simulink model "Teste"  (R2020b)
settings: Solver=VariableStepAuto  StartTime=0.0  StopTime=10.0  RelTol=1e-3
undefined symbols (not defined in the file or in its folder): des, SELECT, T
libraries: simulink x8
(part 2 of 3)

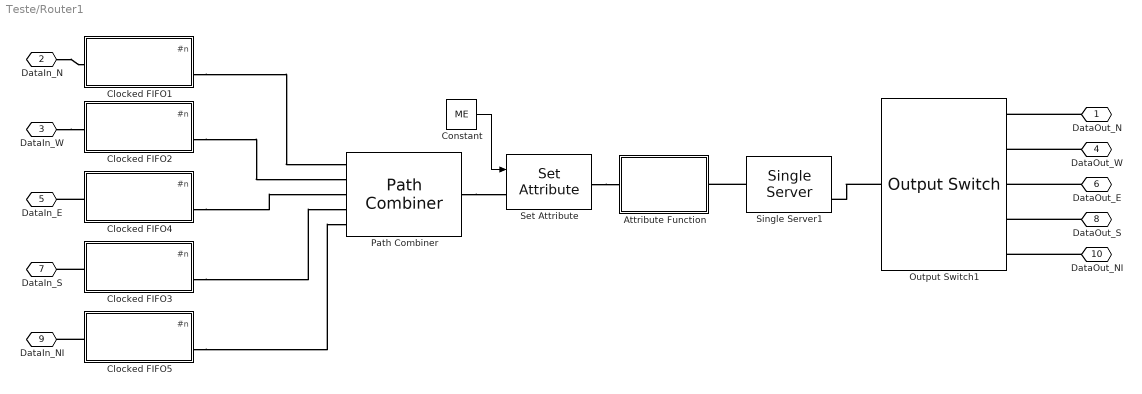
== system Teste/Router1 ==
  Attribute Function : Subsystem  LoadFcn=des.afb.attributefunction_support(gcb,'LoadFcn');  StartFcn=des.afb.attributefunction_support(gcb,'StartFcn');  mask(Attribute Function){OutputNamePrefix=out_}
      mask prompts: OutputNamePrefix "Prefix name"
      settings: CopyFcn=des.afb.attributefunction_support(gcb,'CopyFcn');  OpenFcn=des.afb.attributefunction_support(gcb,'OpenFcn');  ErrorFcn=des.afb.error_redirect
      mask Help: slhelp(gcbh)
      mask Display: image(des_iconLoad('attribFunction.jpg'),'center');
  Clocked FIFO1 : Subsystem  mask{E=1/F, S=S, F=C}
      mask prompts: E "Clock Period (s)"; S "Standard Deviation"; F "FIFO capacity"
  Clocked FIFO2 : Subsystem  mask{E=1, S=.1, F=8}
      mask prompts: E "Clock Period (s)"; S "Standard Deviation"; F "FIFO capacity"
  Clocked FIFO3 : Subsystem  mask{E=1, S=.1, F=8}
      mask prompts: E "Clock Period (s)"; S "Standard Deviation"; F "FIFO capacity"
  Clocked FIFO4 : Subsystem  mask{E=1, S=.1, F=8}
      mask prompts: E "Clock Period (s)"; S "Standard Deviation"; F "FIFO capacity"
  Clocked FIFO5 : Subsystem  mask{E=1, S=.1, F=8}
      mask prompts: E "Clock Period (s)"; S "Standard Deviation"; F "FIFO capacity"
  Constant : Constant  Value=ME
  Output Switch1 : OutputSwitch  NumberOutputPorts=5  SwitchingCriterion=From attribute  AttributeName=RT  InitialConditionsOpt=on  InitialConditions=5
  Path Combiner : PathCombiner  NumberInputPorts=5  InputPortPrecedence=Equiprobable  InitialSeed=2
  Set Attribute : SetAttribute  AttributeName=ME  AttributeFrom=Signal port  EvaluatedAttributeValue={ []}
  Single Server1 : SingleServer  ServiceTime=D  StatNumberDeparted=on
  DataOut_N : PMIOPort  Side=Left
  DataIn_N : PMIOPort  Port=2  Side=Right
  DataIn_W : PMIOPort  Port=3  Side=Left
  DataOut_W : PMIOPort  Port=4  Side=Right
  DataIn_E : PMIOPort  Port=5  Side=Left
  DataOut_E : PMIOPort  Port=6  Side=Right
  DataIn_S : PMIOPort  Port=7  Side=Left
  DataOut_S : PMIOPort  Port=8  Side=Right
  DataIn_NI : PMIOPort  Port=9  Side=Left
  DataOut_NI : PMIOPort  Port=10  Side=Right
  wires:
  Constant/1 -> Set Attribute/1
  connections:
  DataOut_NI/RConn1 -- Output Switch1/RConn5
  DataOut_S/RConn1 -- Output Switch1/RConn4
  DataOut_E/RConn1 -- Output Switch1/RConn3
  DataOut_W/RConn1 -- Output Switch1/RConn2
  DataOut_N/RConn1 -- Output Switch1/RConn1
  Clocked FIFO5/RConn1 -- Path Combiner/LConn5
  Clocked FIFO3/RConn1 -- Path Combiner/LConn4
  Clocked FIFO4/RConn1 -- Path Combiner/LConn3
  Clocked FIFO2/RConn1 -- Path Combiner/LConn2
  Clocked FIFO1/RConn1 -- Path Combiner/LConn1
  Path Combiner/RConn1 -- Set Attribute/LConn1
  Single Server1/LConn1 -- Attribute Function/RConn1
  Output Switch1/LConn1 -- Single Server1/RConn1
  Set Attribute/RConn1 -- Attribute Function/LConn1
  Clocked FIFO5/LConn1 -- DataIn_NI/RConn1
  DataIn_N/RConn1 -- Clocked FIFO1/LConn1
  Clocked FIFO3/LConn1 -- DataIn_S/RConn1
  Clocked FIFO4/LConn1 -- DataIn_E/RConn1
  DataIn_W/RConn1 -- Clocked FIFO2/LConn1

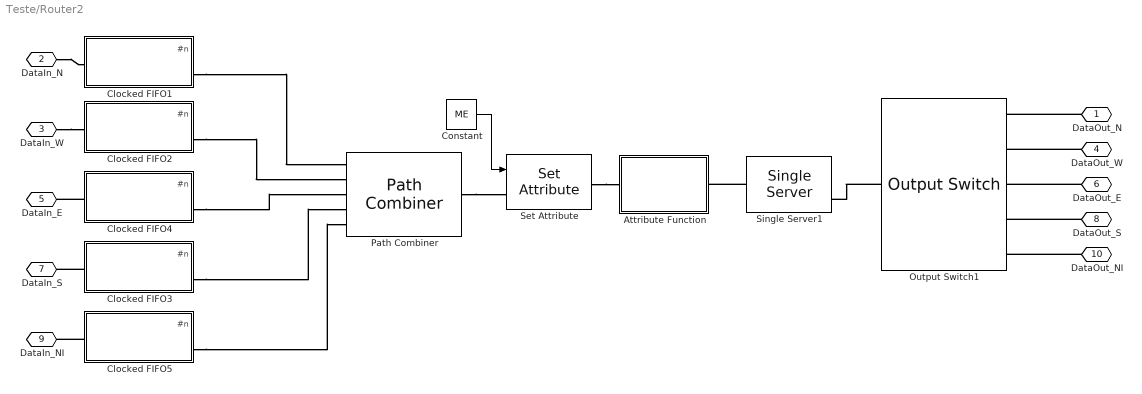
== system Teste/Router2 ==
  Attribute Function : Subsystem  LoadFcn=des.afb.attributefunction_support(gcb,'LoadFcn');  StartFcn=des.afb.attributefunction_support(gcb,'StartFcn');  mask(Attribute Function){OutputNamePrefix=out_}
      mask prompts: OutputNamePrefix "Prefix name"
      settings: CopyFcn=des.afb.attributefunction_support(gcb,'CopyFcn');  OpenFcn=des.afb.attributefunction_support(gcb,'OpenFcn');  ErrorFcn=des.afb.error_redirect
      mask Help: slhelp(gcbh)
      mask Display: image(des_iconLoad('attribFunction.jpg'),'center');
  Clocked FIFO1 : Subsystem  mask{E=1/F, S=S, F=C}
      mask prompts: E "Clock Period (s)"; S "Standard Deviation"; F "FIFO capacity"
  Clocked FIFO2 : Subsystem  mask{E=1, S=.1, F=8}
      mask prompts: E "Clock Period (s)"; S "Standard Deviation"; F "FIFO capacity"
  Clocked FIFO3 : Subsystem  mask{E=1, S=.1, F=8}
      mask prompts: E "Clock Period (s)"; S "Standard Deviation"; F "FIFO capacity"
  Clocked FIFO4 : Subsystem  mask{E=1, S=.1, F=8}
      mask prompts: E "Clock Period (s)"; S "Standard Deviation"; F "FIFO capacity"
  Clocked FIFO5 : Subsystem  mask{E=1, S=.1, F=8}
      mask prompts: E "Clock Period (s)"; S "Standard Deviation"; F "FIFO capacity"
  Constant : Constant  Value=ME
  Output Switch1 : OutputSwitch  NumberOutputPorts=5  SwitchingCriterion=From attribute  AttributeName=RT  InitialConditionsOpt=on  InitialConditions=5
  Path Combiner : PathCombiner  NumberInputPorts=5  InputPortPrecedence=Equiprobable  InitialSeed=2
  Set Attribute : SetAttribute  AttributeName=ME  AttributeFrom=Signal port  EvaluatedAttributeValue={ []}
  Single Server1 : SingleServer  ServiceTime=D  StatNumberDeparted=on
  DataOut_N : PMIOPort  Side=Left
  DataIn_N : PMIOPort  Port=2  Side=Right
  DataIn_W : PMIOPort  Port=3  Side=Left
  DataOut_W : PMIOPort  Port=4  Side=Right
  DataIn_E : PMIOPort  Port=5  Side=Left
  DataOut_E : PMIOPort  Port=6  Side=Right
  DataIn_S : PMIOPort  Port=7  Side=Left
  DataOut_S : PMIOPort  Port=8  Side=Right
  DataIn_NI : PMIOPort  Port=9  Side=Left
  DataOut_NI : PMIOPort  Port=10  Side=Right
  wires:
  Constant/1 -> Set Attribute/1
  connections:
  DataOut_NI/RConn1 -- Output Switch1/RConn5
  DataOut_S/RConn1 -- Output Switch1/RConn4
  DataOut_E/RConn1 -- Output Switch1/RConn3
  DataOut_W/RConn1 -- Output Switch1/RConn2
  DataOut_N/RConn1 -- Output Switch1/RConn1
  Clocked FIFO5/RConn1 -- Path Combiner/LConn5
  Clocked FIFO3/RConn1 -- Path Combiner/LConn4
  Clocked FIFO4/RConn1 -- Path Combiner/LConn3
  Clocked FIFO2/RConn1 -- Path Combiner/LConn2
  Clocked FIFO1/RConn1 -- Path Combiner/LConn1
  Path Combiner/RConn1 -- Set Attribute/LConn1
  Single Server1/LConn1 -- Attribute Function/RConn1
  Output Switch1/LConn1 -- Single Server1/RConn1
  Set Attribute/RConn1 -- Attribute Function/LConn1
  Clocked FIFO5/LConn1 -- DataIn_NI/RConn1
  DataIn_N/RConn1 -- Clocked FIFO1/LConn1
  Clocked FIFO3/LConn1 -- DataIn_S/RConn1
  Clocked FIFO4/LConn1 -- DataIn_E/RConn1
  DataIn_W/RConn1 -- Clocked FIFO2/LConn1

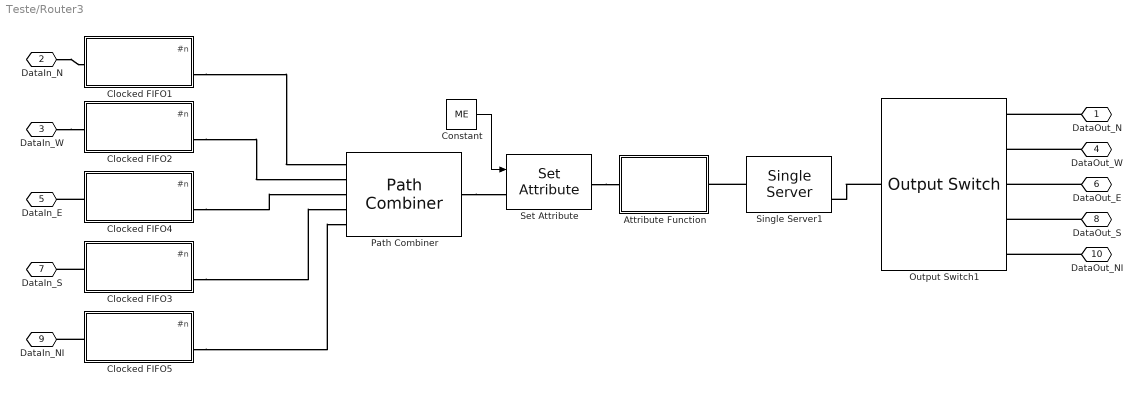
== system Teste/Router3 ==
  Attribute Function : Subsystem  LoadFcn=des.afb.attributefunction_support(gcb,'LoadFcn');  StartFcn=des.afb.attributefunction_support(gcb,'StartFcn');  mask(Attribute Function){OutputNamePrefix=out_}
      mask prompts: OutputNamePrefix "Prefix name"
      settings: CopyFcn=des.afb.attributefunction_support(gcb,'CopyFcn');  OpenFcn=des.afb.attributefunction_support(gcb,'OpenFcn');  ErrorFcn=des.afb.error_redirect
      mask Help: slhelp(gcbh)
      mask Display: image(des_iconLoad('attribFunction.jpg'),'center');
  Clocked FIFO1 : Subsystem  mask{E=1/F, S=S, F=C}
      mask prompts: E "Clock Period (s)"; S "Standard Deviation"; F "FIFO capacity"
  Clocked FIFO2 : Subsystem  mask{E=1, S=.1, F=8}
      mask prompts: E "Clock Period (s)"; S "Standard Deviation"; F "FIFO capacity"
  Clocked FIFO3 : Subsystem  mask{E=1, S=.1, F=8}
      mask prompts: E "Clock Period (s)"; S "Standard Deviation"; F "FIFO capacity"
  Clocked FIFO4 : Subsystem  mask{E=1, S=.1, F=8}
      mask prompts: E "Clock Period (s)"; S "Standard Deviation"; F "FIFO capacity"
  Clocked FIFO5 : Subsystem  mask{E=1, S=.1, F=8}
      mask prompts: E "Clock Period (s)"; S "Standard Deviation"; F "FIFO capacity"
  Constant : Constant  Value=ME
  Output Switch1 : OutputSwitch  NumberOutputPorts=5  SwitchingCriterion=From attribute  AttributeName=RT  InitialConditionsOpt=on  InitialConditions=5
  Path Combiner : PathCombiner  NumberInputPorts=5  InputPortPrecedence=Equiprobable  InitialSeed=2
  Set Attribute : SetAttribute  AttributeName=ME  AttributeFrom=Signal port  EvaluatedAttributeValue={ []}
  Single Server1 : SingleServer  ServiceTime=D  StatNumberDeparted=on
  DataOut_N : PMIOPort  Side=Left
  DataIn_N : PMIOPort  Port=2  Side=Right
  DataIn_W : PMIOPort  Port=3  Side=Left
  DataOut_W : PMIOPort  Port=4  Side=Right
  DataIn_E : PMIOPort  Port=5  Side=Left
  DataOut_E : PMIOPort  Port=6  Side=Right
  DataIn_S : PMIOPort  Port=7  Side=Left
  DataOut_S : PMIOPort  Port=8  Side=Right
  DataIn_NI : PMIOPort  Port=9  Side=Left
  DataOut_NI : PMIOPort  Port=10  Side=Right
  wires:
  Constant/1 -> Set Attribute/1
  connections:
  DataOut_NI/RConn1 -- Output Switch1/RConn5
  DataOut_S/RConn1 -- Output Switch1/RConn4
  DataOut_E/RConn1 -- Output Switch1/RConn3
  DataOut_W/RConn1 -- Output Switch1/RConn2
  DataOut_N/RConn1 -- Output Switch1/RConn1
  Clocked FIFO5/RConn1 -- Path Combiner/LConn5
  Clocked FIFO3/RConn1 -- Path Combiner/LConn4
  Clocked FIFO4/RConn1 -- Path Combiner/LConn3
  Clocked FIFO2/RConn1 -- Path Combiner/LConn2
  Clocked FIFO1/RConn1 -- Path Combiner/LConn1
  Path Combiner/RConn1 -- Set Attribute/LConn1
  Single Server1/LConn1 -- Attribute Function/RConn1
  Output Switch1/LConn1 -- Single Server1/RConn1
  Set Attribute/RConn1 -- Attribute Function/LConn1
  Clocked FIFO5/LConn1 -- DataIn_NI/RConn1
  DataIn_N/RConn1 -- Clocked FIFO1/LConn1
  Clocked FIFO3/LConn1 -- DataIn_S/RConn1
  Clocked FIFO4/LConn1 -- DataIn_E/RConn1
  DataIn_W/RConn1 -- Clocked FIFO2/LConn1

== system Teste/Router4 ==
  Attribute Function : Subsystem  LoadFcn=des.afb.attributefunction_support(gcb,'LoadFcn');  StartFcn=des.afb.attributefunction_support(gcb,'StartFcn');  mask(Attribute Function){OutputNamePrefix=out_}
      mask prompts: OutputNamePrefix "Prefix name"
      settings: CopyFcn=des.afb.attributefunction_support(gcb,'CopyFcn');  OpenFcn=des.afb.attributefunction_support(gcb,'OpenFcn');  ErrorFcn=des.afb.error_redirect
      mask Help: slhelp(gcbh)
      mask Display: image(des_iconLoad('attribFunction.jpg'),'center');
  Clocked FIFO1 : Subsystem  mask{E=1/F, S=S, F=C}
      mask prompts: E "Clock Period (s)"; S "Standard Deviation"; F "FIFO capacity"
  Clocked FIFO2 : Subsystem  mask{E=1, S=.1, F=8}
      mask prompts: E "Clock Period (s)"; S "Standard Deviation"; F "FIFO capacity"
  Clocked FIFO3 : Subsystem  mask{E=1, S=.1, F=8}
      mask prompts: E "Clock Period (s)"; S "Standard Deviation"; F "FIFO capacity"
  Clocked FIFO4 : Subsystem  mask{E=1, S=.1, F=8}
      mask prompts: E "Clock Period (s)"; S "Standard Deviation"; F "FIFO capacity"
  Clocked FIFO5 : Subsystem  mask{E=1, S=.1, F=8}
      mask prompts: E "Clock Period (s)"; S "Standard Deviation"; F "FIFO capacity"
  Constant : Constant  Value=ME
  Output Switch1 : OutputSwitch  NumberOutputPorts=5  SwitchingCriterion=From attribute  AttributeName=RT  InitialConditionsOpt=on  InitialConditions=5
  Path Combiner : PathCombiner  NumberInputPorts=5  InputPortPrecedence=Equiprobable  InitialSeed=2
  Set Attribute : SetAttribute  AttributeName=ME  AttributeFrom=Signal port  EvaluatedAttributeValue={ []}
  Single Server1 : SingleServer  ServiceTime=D  StatNumberDeparted=on
  DataOut_N : PMIOPort  Side=Left
  DataIn_N : PMIOPort  Port=2  Side=Right
  DataIn_W : PMIOPort  Port=3  Side=Left
  DataOut_W : PMIOPort  Port=4  Side=Right
  DataIn_E : PMIOPort  Port=5  Side=Left
  DataOut_E : PMIOPort  Port=6  Side=Right
  DataIn_S : PMIOPort  Port=7  Side=Left
  DataOut_S : PMIOPort  Port=8  Side=Right
  DataIn_NI : PMIOPort  Port=9  Side=Left
  DataOut_NI : PMIOPort  Port=10  Side=Right
  wires:
  Constant/1 -> Set Attribute/1
  connections:
  DataOut_NI/RConn1 -- Output Switch1/RConn5
  DataOut_S/RConn1 -- Output Switch1/RConn4
  DataOut_E/RConn1 -- Output Switch1/RConn3
  DataOut_W/RConn1 -- Output Switch1/RConn2
  DataOut_N/RConn1 -- Output Switch1/RConn1
  Clocked FIFO5/RConn1 -- Path Combiner/LConn5
  Clocked FIFO3/RConn1 -- Path Combiner/LConn4
  Clocked FIFO4/RConn1 -- Path Combiner/LConn3
  Clocked FIFO2/RConn1 -- Path Combiner/LConn2
  Clocked FIFO1/RConn1 -- Path Combiner/LConn1
  Path Combiner/RConn1 -- Set Attribute/LConn1
  Single Server1/LConn1 -- Attribute Function/RConn1
  Output Switch1/LConn1 -- Single Server1/RConn1
  Set Attribute/RConn1 -- Attribute Function/LConn1
  Clocked FIFO5/LConn1 -- DataIn_NI/RConn1
  DataIn_N/RConn1 -- Clocked FIFO1/LConn1
  Clocked FIFO3/LConn1 -- DataIn_S/RConn1
  Clocked FIFO4/LConn1 -- DataIn_E/RConn1
  DataIn_W/RConn1 -- Clocked FIFO2/LConn1

== system Teste/Router5 ==
  Attribute Function : Subsystem  LoadFcn=des.afb.attributefunction_support(gcb,'LoadFcn');  StartFcn=des.afb.attributefunction_support(gcb,'StartFcn');  mask(Attribute Function){OutputNamePrefix=out_}
      mask prompts: OutputNamePrefix "Prefix name"
      settings: CopyFcn=des.afb.attributefunction_support(gcb,'CopyFcn');  OpenFcn=des.afb.attributefunction_support(gcb,'OpenFcn');  ErrorFcn=des.afb.error_redirect
      mask Help: slhelp(gcbh)
      mask Display: image(des_iconLoad('attribFunction.jpg'),'center');
  Clocked FIFO1 : Subsystem  mask{E=1/F, S=S, F=C}
      mask prompts: E "Clock Period (s)"; S "Standard Deviation"; F "FIFO capacity"
  Clocked FIFO2 : Subsystem  mask{E=1, S=.1, F=8}
      mask prompts: E "Clock Period (s)"; S "Standard Deviation"; F "FIFO capacity"
  Clocked FIFO3 : Subsystem  mask{E=1, S=.1, F=8}
      mask prompts: E "Clock Period (s)"; S "Standard Deviation"; F "FIFO capacity"
  Clocked FIFO4 : Subsystem  mask{E=1, S=.1, F=8}
      mask prompts: E "Clock Period (s)"; S "Standard Deviation"; F "FIFO capacity"
  Clocked FIFO5 : Subsystem  mask{E=1, S=.1, F=8}
      mask prompts: E "Clock Period (s)"; S "Standard Deviation"; F "FIFO capacity"
  Constant : Constant  Value=ME
  Output Switch1 : OutputSwitch  NumberOutputPorts=5  SwitchingCriterion=From attribute  AttributeName=RT  InitialConditionsOpt=on  InitialConditions=5
  Path Combiner : PathCombiner  NumberInputPorts=5  InputPortPrecedence=Equiprobable  InitialSeed=2
  Set Attribute : SetAttribute  AttributeName=ME  AttributeFrom=Signal port  EvaluatedAttributeValue={ []}
  Single Server1 : SingleServer  ServiceTime=D  StatNumberDeparted=on
  DataOut_N : PMIOPort  Side=Left
  DataIn_N : PMIOPort  Port=2  Side=Right
  DataIn_W : PMIOPort  Port=3  Side=Left
  DataOut_W : PMIOPort  Port=4  Side=Right
  DataIn_E : PMIOPort  Port=5  Side=Left
  DataOut_E : PMIOPort  Port=6  Side=Right
  DataIn_S : PMIOPort  Port=7  Side=Left
  DataOut_S : PMIOPort  Port=8  Side=Right
  DataIn_NI : PMIOPort  Port=9  Side=Left
  DataOut_NI : PMIOPort  Port=10  Side=Right
  wires:
  Constant/1 -> Set Attribute/1
  connections:
  DataOut_NI/RConn1 -- Output Switch1/RConn5
  DataOut_S/RConn1 -- Output Switch1/RConn4
  DataOut_E/RConn1 -- Output Switch1/RConn3
  DataOut_W/RConn1 -- Output Switch1/RConn2
  DataOut_N/RConn1 -- Output Switch1/RConn1
  Clocked FIFO5/RConn1 -- Path Combiner/LConn5
  Clocked FIFO3/RConn1 -- Path Combiner/LConn4
  Clocked FIFO4/RConn1 -- Path Combiner/LConn3
  Clocked FIFO2/RConn1 -- Path Combiner/LConn2
  Clocked FIFO1/RConn1 -- Path Combiner/LConn1
  Path Combiner/RConn1 -- Set Attribute/LConn1
  Single Server1/LConn1 -- Attribute Function/RConn1
  Output Switch1/LConn1 -- Single Server1/RConn1
  Set Attribute/RConn1 -- Attribute Function/LConn1
  Clocked FIFO5/LConn1 -- DataIn_NI/RConn1
  DataIn_N/RConn1 -- Clocked FIFO1/LConn1
  Clocked FIFO3/LConn1 -- DataIn_S/RConn1
  Clocked FIFO4/LConn1 -- DataIn_E/RConn1
  DataIn_W/RConn1 -- Clocked FIFO2/LConn1

== system Teste/Router6 ==
  Attribute Function : Subsystem  LoadFcn=des.afb.attributefunction_support(gcb,'LoadFcn');  StartFcn=des.afb.attributefunction_support(gcb,'StartFcn');  mask(Attribute Function){OutputNamePrefix=out_}
      mask prompts: OutputNamePrefix "Prefix name"
      settings: CopyFcn=des.afb.attributefunction_support(gcb,'CopyFcn');  OpenFcn=des.afb.attributefunction_support(gcb,'OpenFcn');  ErrorFcn=des.afb.error_redirect
      mask Help: slhelp(gcbh)
      mask Display: image(des_iconLoad('attribFunction.jpg'),'center');
  Clocked FIFO1 : Subsystem  mask{E=1/F, S=S, F=C}
      mask prompts: E "Clock Period (s)"; S "Standard Deviation"; F "FIFO capacity"
  Clocked FIFO2 : Subsystem  mask{E=1, S=.1, F=8}
      mask prompts: E "Clock Period (s)"; S "Standard Deviation"; F "FIFO capacity"
  Clocked FIFO3 : Subsystem  mask{E=1, S=.1, F=8}
      mask prompts: E "Clock Period (s)"; S "Standard Deviation"; F "FIFO capacity"
  Clocked FIFO4 : Subsystem  mask{E=1, S=.1, F=8}
      mask prompts: E "Clock Period (s)"; S "Standard Deviation"; F "FIFO capacity"
  Clocked FIFO5 : Subsystem  mask{E=1, S=.1, F=8}
      mask prompts: E "Clock Period (s)"; S "Standard Deviation"; F "FIFO capacity"
  Constant : Constant  Value=ME
  Output Switch1 : OutputSwitch  NumberOutputPorts=5  SwitchingCriterion=From attribute  AttributeName=RT  InitialConditionsOpt=on  InitialConditions=5
  Path Combiner : PathCombiner  NumberInputPorts=5  InputPortPrecedence=Equiprobable  InitialSeed=2
  Set Attribute : SetAttribute  AttributeName=ME  AttributeFrom=Signal port  EvaluatedAttributeValue={ []}
  Single Server1 : SingleServer  ServiceTime=D  StatNumberDeparted=on
  DataOut_N : PMIOPort  Side=Left
  DataIn_N : PMIOPort  Port=2  Side=Right
  DataIn_W : PMIOPort  Port=3  Side=Left
  DataOut_W : PMIOPort  Port=4  Side=Right
  DataIn_E : PMIOPort  Port=5  Side=Left
  DataOut_E : PMIOPort  Port=6  Side=Right
  DataIn_S : PMIOPort  Port=7  Side=Left
  DataOut_S : PMIOPort  Port=8  Side=Right
  DataIn_NI : PMIOPort  Port=9  Side=Left
  DataOut_NI : PMIOPort  Port=10  Side=Right
  wires:
  Constant/1 -> Set Attribute/1
  connections:
  DataOut_NI/RConn1 -- Output Switch1/RConn5
  DataOut_S/RConn1 -- Output Switch1/RConn4
  DataOut_E/RConn1 -- Output Switch1/RConn3
  DataOut_W/RConn1 -- Output Switch1/RConn2
  DataOut_N/RConn1 -- Output Switch1/RConn1
  Clocked FIFO5/RConn1 -- Path Combiner/LConn5
  Clocked FIFO3/RConn1 -- Path Combiner/LConn4
  Clocked FIFO4/RConn1 -- Path Combiner/LConn3
  Clocked FIFO2/RConn1 -- Path Combiner/LConn2
  Clocked FIFO1/RConn1 -- Path Combiner/LConn1
  Path Combiner/RConn1 -- Set Attribute/LConn1
  Single Server1/LConn1 -- Attribute Function/RConn1
  Output Switch1/LConn1 -- Single Server1/RConn1
  Set Attribute/RConn1 -- Attribute Function/LConn1
  Clocked FIFO5/LConn1 -- DataIn_NI/RConn1
  DataIn_N/RConn1 -- Clocked FIFO1/LConn1
  Clocked FIFO3/LConn1 -- DataIn_S/RConn1
  Clocked FIFO4/LConn1 -- DataIn_E/RConn1
  DataIn_W/RConn1 -- Clocked FIFO2/LConn1

== system Teste/Router7 ==
  Attribute Function : Subsystem  LoadFcn=des.afb.attributefunction_support(gcb,'LoadFcn');  StartFcn=des.afb.attributefunction_support(gcb,'StartFcn');  mask(Attribute Function){OutputNamePrefix=out_}
      mask prompts: OutputNamePrefix "Prefix name"
      settings: CopyFcn=des.afb.attributefunction_support(gcb,'CopyFcn');  OpenFcn=des.afb.attributefunction_support(gcb,'OpenFcn');  ErrorFcn=des.afb.error_redirect
      mask Help: slhelp(gcbh)
      mask Display: image(des_iconLoad('attribFunction.jpg'),'center');
  Clocked FIFO1 : Subsystem  mask{E=1/F, S=S, F=C}
      mask prompts: E "Clock Period (s)"; S "Standard Deviation"; F "FIFO capacity"
  Clocked FIFO2 : Subsystem  mask{E=1, S=.1, F=8}
      mask prompts: E "Clock Period (s)"; S "Standard Deviation"; F "FIFO capacity"
  Clocked FIFO3 : Subsystem  mask{E=1, S=.1, F=8}
      mask prompts: E "Clock Period (s)"; S "Standard Deviation"; F "FIFO capacity"
  Clocked FIFO4 : Subsystem  mask{E=1, S=.1, F=8}
      mask prompts: E "Clock Period (s)"; S "Standard Deviation"; F "FIFO capacity"
  Clocked FIFO5 : Subsystem  mask{E=1, S=.1, F=8}
      mask prompts: E "Clock Period (s)"; S "Standard Deviation"; F "FIFO capacity"
  Constant : Constant  Value=ME
  Output Switch1 : OutputSwitch  NumberOutputPorts=5  SwitchingCriterion=From attribute  AttributeName=RT  InitialConditionsOpt=on  InitialConditions=5
  Path Combiner : PathCombiner  NumberInputPorts=5  InputPortPrecedence=Equiprobable  InitialSeed=2
  Set Attribute : SetAttribute  AttributeName=ME  AttributeFrom=Signal port  EvaluatedAttributeValue={ []}
  Single Server1 : SingleServer  ServiceTime=D  StatNumberDeparted=on
  DataOut_N : PMIOPort  Side=Left
  DataIn_N : PMIOPort  Port=2  Side=Right
  DataIn_W : PMIOPort  Port=3  Side=Left
  DataOut_W : PMIOPort  Port=4  Side=Right
  DataIn_E : PMIOPort  Port=5  Side=Left
  DataOut_E : PMIOPort  Port=6  Side=Right
  DataIn_S : PMIOPort  Port=7  Side=Left
  DataOut_S : PMIOPort  Port=8  Side=Right
  DataIn_NI : PMIOPort  Port=9  Side=Left
  DataOut_NI : PMIOPort  Port=10  Side=Right
  wires:
  Constant/1 -> Set Attribute/1
  connections:
  DataOut_NI/RConn1 -- Output Switch1/RConn5
  DataOut_S/RConn1 -- Output Switch1/RConn4
  DataOut_E/RConn1 -- Output Switch1/RConn3
  DataOut_W/RConn1 -- Output Switch1/RConn2
  DataOut_N/RConn1 -- Output Switch1/RConn1
  Clocked FIFO5/RConn1 -- Path Combiner/LConn5
  Clocked FIFO3/RConn1 -- Path Combiner/LConn4
  Clocked FIFO4/RConn1 -- Path Combiner/LConn3
  Clocked FIFO2/RConn1 -- Path Combiner/LConn2
  Clocked FIFO1/RConn1 -- Path Combiner/LConn1
  Path Combiner/RConn1 -- Set Attribute/LConn1
  Single Server1/LConn1 -- Attribute Function/RConn1
  Output Switch1/LConn1 -- Single Server1/RConn1
  Set Attribute/RConn1 -- Attribute Function/LConn1
  Clocked FIFO5/LConn1 -- DataIn_NI/RConn1
  DataIn_N/RConn1 -- Clocked FIFO1/LConn1
  Clocked FIFO3/LConn1 -- DataIn_S/RConn1
  Clocked FIFO4/LConn1 -- DataIn_E/RConn1
  DataIn_W/RConn1 -- Clocked FIFO2/LConn1

== system Teste/Router8 ==
  Attribute Function : Subsystem  LoadFcn=des.afb.attributefunction_support(gcb,'LoadFcn');  StartFcn=des.afb.attributefunction_support(gcb,'StartFcn');  mask(Attribute Function){OutputNamePrefix=out_}
      mask prompts: OutputNamePrefix "Prefix name"
      settings: CopyFcn=des.afb.attributefunction_support(gcb,'CopyFcn');  OpenFcn=des.afb.attributefunction_support(gcb,'OpenFcn');  ErrorFcn=des.afb.error_redirect
      mask Help: slhelp(gcbh)
      mask Display: image(des_iconLoad('attribFunction.jpg'),'center');
  Clocked FIFO1 : Subsystem  mask{E=1/F, S=S, F=C}
      mask prompts: E "Clock Period (s)"; S "Standard Deviation"; F "FIFO capacity"
  Clocked FIFO2 : Subsystem  mask{E=1, S=.1, F=8}
      mask prompts: E "Clock Period (s)"; S "Standard Deviation"; F "FIFO capacity"
  Clocked FIFO3 : Subsystem  mask{E=1, S=.1, F=8}
      mask prompts: E "Clock Period (s)"; S "Standard Deviation"; F "FIFO capacity"
  Clocked FIFO4 : Subsystem  mask{E=1, S=.1, F=8}
      mask prompts: E "Clock Period (s)"; S "Standard Deviation"; F "FIFO capacity"
  Clocked FIFO5 : Subsystem  mask{E=1, S=.1, F=8}
      mask prompts: E "Clock Period (s)"; S "Standard Deviation"; F "FIFO capacity"
  Constant : Constant  Value=ME
  Output Switch1 : OutputSwitch  NumberOutputPorts=5  SwitchingCriterion=From attribute  AttributeName=RT  InitialConditionsOpt=on  InitialConditions=5
  Path Combiner : PathCombiner  NumberInputPorts=5  InputPortPrecedence=Equiprobable  InitialSeed=2
  Set Attribute : SetAttribute  AttributeName=ME  AttributeFrom=Signal port  EvaluatedAttributeValue={ []}
  Single Server1 : SingleServer  ServiceTime=D  StatNumberDeparted=on
  DataOut_N : PMIOPort  Side=Left
  DataIn_N : PMIOPort  Port=2  Side=Right
  DataIn_W : PMIOPort  Port=3  Side=Left
  DataOut_W : PMIOPort  Port=4  Side=Right
  DataIn_E : PMIOPort  Port=5  Side=Left
  DataOut_E : PMIOPort  Port=6  Side=Right
  DataIn_S : PMIOPort  Port=7  Side=Left
  DataOut_S : PMIOPort  Port=8  Side=Right
  DataIn_NI : PMIOPort  Port=9  Side=Left
  DataOut_NI : PMIOPort  Port=10  Side=Right
  wires:
  Constant/1 -> Set Attribute/1
  connections:
  DataOut_NI/RConn1 -- Output Switch1/RConn5
  DataOut_S/RConn1 -- Output Switch1/RConn4
  DataOut_E/RConn1 -- Output Switch1/RConn3
  DataOut_W/RConn1 -- Output Switch1/RConn2
  DataOut_N/RConn1 -- Output Switch1/RConn1
  Clocked FIFO5/RConn1 -- Path Combiner/LConn5
  Clocked FIFO3/RConn1 -- Path Combiner/LConn4
  Clocked FIFO4/RConn1 -- Path Combiner/LConn3
  Clocked FIFO2/RConn1 -- Path Combiner/LConn2
  Clocked FIFO1/RConn1 -- Path Combiner/LConn1
  Path Combiner/RConn1 -- Set Attribute/LConn1
  Single Server1/LConn1 -- Attribute Function/RConn1
  Output Switch1/LConn1 -- Single Server1/RConn1
  Set Attribute/RConn1 -- Attribute Function/LConn1
  Clocked FIFO5/LConn1 -- DataIn_NI/RConn1
  DataIn_N/RConn1 -- Clocked FIFO1/LConn1
  Clocked FIFO3/LConn1 -- DataIn_S/RConn1
  Clocked FIFO4/LConn1 -- DataIn_E/RConn1
  DataIn_W/RConn1 -- Clocked FIFO2/LConn1

== system Teste/PE1/Create Generator Selection Variable ==
  function : TriggerPort  TriggerType=function-call  VariantControl=(inherit)
  Repeating Sequence Stair : simulink/Sources/Repeating Sequence Stair  OutValues=[0 1].'  tsamp=-1  OutMin=[]  OutMax=[]  OutDataTypeStr=float('double')  OutputDataTypeScalingMode=Specify via dialog  OutDataType=float('double')  ConRadixGroup=Best Precision: Vector-wise  OutScaling=2^-12
  Out1 : Outport
  wires:
  Repeating Sequence Stair/1 -> Out1/1

== system Teste/PE2/Create Generator Selection Variable ==
  function : TriggerPort  TriggerType=function-call  VariantControl=(inherit)
  Repeating Sequence Stair : simulink/Sources/Repeating Sequence Stair  OutValues=[0 1].'  tsamp=-1  OutMin=[]  OutMax=[]  OutDataTypeStr=float('double')  OutputDataTypeScalingMode=Specify via dialog  OutDataType=float('double')  ConRadixGroup=Best Precision: Vector-wise  OutScaling=2^-12
  Out1 : Outport
  wires:
  Repeating Sequence Stair/1 -> Out1/1

== system Teste/PE3/Create Generator Selection Variable ==
  function : TriggerPort  TriggerType=function-call  VariantControl=(inherit)
  Repeating Sequence Stair : simulink/Sources/Repeating Sequence Stair  OutValues=[0 1].'  tsamp=-1  OutMin=[]  OutMax=[]  OutDataTypeStr=float('double')  OutputDataTypeScalingMode=Specify via dialog  OutDataType=float('double')  ConRadixGroup=Best Precision: Vector-wise  OutScaling=2^-12
  Out1 : Outport
  wires:
  Repeating Sequence Stair/1 -> Out1/1

== system Teste/PE4/Create Generator Selection Variable ==
  function : TriggerPort  TriggerType=function-call  VariantControl=(inherit)
  Repeating Sequence Stair : simulink/Sources/Repeating Sequence Stair  OutValues=[0 1].'  tsamp=-1  OutMin=[]  OutMax=[]  OutDataTypeStr=float('double')  OutputDataTypeScalingMode=Specify via dialog  OutDataType=float('double')  ConRadixGroup=Best Precision: Vector-wise  OutScaling=2^-12
  Out1 : Outport
  wires:
  Repeating Sequence Stair/1 -> Out1/1

== system Teste/PE5/Create Generator Selection Variable ==
  function : TriggerPort  TriggerType=function-call  VariantControl=(inherit)
  Repeating Sequence Stair : simulink/Sources/Repeating Sequence Stair  OutValues=[0 1].'  tsamp=-1  OutMin=[]  OutMax=[]  OutDataTypeStr=float('double')  OutputDataTypeScalingMode=Specify via dialog  OutDataType=float('double')  ConRadixGroup=Best Precision: Vector-wise  OutScaling=2^-12
  Out1 : Outport
  wires:
  Repeating Sequence Stair/1 -> Out1/1

== system Teste/PE6/Create Generator Selection Variable ==
  function : TriggerPort  TriggerType=function-call  VariantControl=(inherit)
  Repeating Sequence Stair : simulink/Sources/Repeating Sequence Stair  OutValues=[0 1].'  tsamp=-1  OutMin=[]  OutMax=[]  OutDataTypeStr=float('double')  OutputDataTypeScalingMode=Specify via dialog  OutDataType=float('double')  ConRadixGroup=Best Precision: Vector-wise  OutScaling=2^-12
  Out1 : Outport
  wires:
  Repeating Sequence Stair/1 -> Out1/1

== system Teste/PE7/Create Generator Selection Variable ==
  function : TriggerPort  TriggerType=function-call  VariantControl=(inherit)
  Repeating Sequence Stair : simulink/Sources/Repeating Sequence Stair  OutValues=[0 1].'  tsamp=-1  OutMin=[]  OutMax=[]  OutDataTypeStr=float('double')  OutputDataTypeScalingMode=Specify via dialog  OutDataType=float('double')  ConRadixGroup=Best Precision: Vector-wise  OutScaling=2^-12
  Out1 : Outport
  wires:
  Repeating Sequence Stair/1 -> Out1/1

== system Teste/PE8/Create Generator Selection Variable ==
  function : TriggerPort  TriggerType=function-call  VariantControl=(inherit)
  Repeating Sequence Stair : simulink/Sources/Repeating Sequence Stair  OutValues=[0 1].'  tsamp=-1  OutMin=[]  OutMax=[]  OutDataTypeStr=float('double')  OutputDataTypeScalingMode=Specify via dialog  OutDataType=float('double')  ConRadixGroup=Best Precision: Vector-wise  OutScaling=2^-12
  Out1 : Outport
  wires:
  Repeating Sequence Stair/1 -> Out1/1

== system Teste/Router1/Attribute Function ==
  MATLAB Function : MATLAB Function  TreatAsAtomicUnit=on
  __DMLF__EDE2FCE__ : EntityDepartureFunctionCallGenerator  TimingFunctionCallF1=Before entity departure  IsInsideAFB=on
  __DMLF__GA__ : GetAttribute  AttributeName=DST|ME  AttributeMissing=Error|Error  AttributeDefaultValue=1|1  AttributeTreatAsVector=1|1  AttributeSendTiming=Before entity departure|Before entity departure  EvaluatedDefaultAttributeValue={ [];[]}  IsInsideAFB=on
      settings: OutputPortMap=o1,o2
  __DMLF__SA__ : SetAttribute  AttributeName=RT  AttributeFrom=Signal port  EvaluatedAttributeValue={ []}  IsInsideAFB=on
  IN : PMIOPort  Side=Left
  OUT : PMIOPort  Port=2  Side=Right
  wires:
  MATLAB Function/1(out_RT) -> __DMLF__SA__/1
  __DMLF__GA__/2 -> MATLAB Function/2(ME)
  __DMLF__GA__/1 -> MATLAB Function/1(DST)
  __DMLF__EDE2FCE__/1 -> MATLAB Function/Trigger
  connections:
  __DMLF__SA__/RConn1 -- OUT/RConn1
  IN/RConn1 -- __DMLF__GA__/LConn1
  __DMLF__GA__/RConn1 -- __DMLF__EDE2FCE__/LConn1
  __DMLF__SA__/LConn1 -- __DMLF__EDE2FCE__/RConn1

== system Teste/Router1/Clocked FIFO1 ==
  Event-Based Random Number : EventBasedRandomNumber  Distribution=Gaussian (normal)  meanNorm=E  stdNorm=S
  FIFO Queue : FIFOQueue  Capacity=F  StatNumberInBlock=on
      settings: OutputPortMap=o1
  Release Gate : ReleaseGate  OpenGateUpon=Function call from port fcn
  Time-Based Function-Call Generator : TimeBasedFunctionCallGenerator  EventGenerationMode=Period from port  Period=T
  Input : PMIOPort  Side=Left
  Output : PMIOPort  Port=2  Side=Right
  #n : Outport
  wires:
  Event-Based Random Number/1 -> Time-Based Function-Call Generator/1
  FIFO Queue/1 -> #n/1
  Time-Based Function-Call Generator/1 -> Release Gate/1
  connections:
  FIFO Queue/RConn1 -- Release Gate/LConn1
  Release Gate/RConn1 -- Output/RConn1
  FIFO Queue/LConn1 -- Input/RConn1

== system Teste/Router1/Clocked FIFO2 ==
  Event-Based Random Number : EventBasedRandomNumber  Distribution=Gaussian (normal)  meanNorm=E  stdNorm=S
  FIFO Queue : FIFOQueue  Capacity=F  StatNumberInBlock=on
      settings: OutputPortMap=o1
  Release Gate : ReleaseGate  OpenGateUpon=Function call from port fcn
  Time-Based Function-Call Generator : TimeBasedFunctionCallGenerator  EventGenerationMode=Period from port  Period=T
  Input : PMIOPort  Side=Left
  Output : PMIOPort  Port=2  Side=Right
  #n : Outport
  wires:
  Event-Based Random Number/1 -> Time-Based Function-Call Generator/1
  FIFO Queue/1 -> #n/1
  Time-Based Function-Call Generator/1 -> Release Gate/1
  connections:
  FIFO Queue/RConn1 -- Release Gate/LConn1
  Release Gate/RConn1 -- Output/RConn1
  FIFO Queue/LConn1 -- Input/RConn1

== system Teste/Router1/Clocked FIFO3 ==
  Event-Based Random Number : EventBasedRandomNumber  Distribution=Gaussian (normal)  meanNorm=E  stdNorm=S
  FIFO Queue : FIFOQueue  Capacity=F  StatNumberInBlock=on
      settings: OutputPortMap=o1
  Release Gate : ReleaseGate  OpenGateUpon=Function call from port fcn
  Time-Based Function-Call Generator : TimeBasedFunctionCallGenerator  EventGenerationMode=Period from port  Period=T
  Input : PMIOPort  Side=Left
  Output : PMIOPort  Port=2  Side=Right
  #n : Outport
  wires:
  Event-Based Random Number/1 -> Time-Based Function-Call Generator/1
  FIFO Queue/1 -> #n/1
  Time-Based Function-Call Generator/1 -> Release Gate/1
  connections:
  FIFO Queue/RConn1 -- Release Gate/LConn1
  Release Gate/RConn1 -- Output/RConn1
  FIFO Queue/LConn1 -- Input/RConn1

== system Teste/Router1/Clocked FIFO4 ==
  Event-Based Random Number : EventBasedRandomNumber  Distribution=Gaussian (normal)  meanNorm=E  stdNorm=S
  FIFO Queue : FIFOQueue  Capacity=F  StatNumberInBlock=on
      settings: OutputPortMap=o1
  Release Gate : ReleaseGate  OpenGateUpon=Function call from port fcn
  Time-Based Function-Call Generator : TimeBasedFunctionCallGenerator  EventGenerationMode=Period from port  Period=T
  Input : PMIOPort  Side=Left
  Output : PMIOPort  Port=2  Side=Right
  #n : Outport
  wires:
  Event-Based Random Number/1 -> Time-Based Function-Call Generator/1
  FIFO Queue/1 -> #n/1
  Time-Based Function-Call Generator/1 -> Release Gate/1
  connections:
  FIFO Queue/RConn1 -- Release Gate/LConn1
  Release Gate/RConn1 -- Output/RConn1
  FIFO Queue/LConn1 -- Input/RConn1

== system Teste/Router1/Clocked FIFO5 ==
  Event-Based Random Number : EventBasedRandomNumber  Distribution=Gaussian (normal)  meanNorm=E  stdNorm=S
  FIFO Queue : FIFOQueue  Capacity=F  StatNumberInBlock=on
      settings: OutputPortMap=o1
  Release Gate : ReleaseGate  OpenGateUpon=Function call from port fcn
  Time-Based Function-Call Generator : TimeBasedFunctionCallGenerator  EventGenerationMode=Period from port  Period=T
  Input : PMIOPort  Side=Left
  Output : PMIOPort  Port=2  Side=Right
  #n : Outport
  wires:
  Event-Based Random Number/1 -> Time-Based Function-Call Generator/1
  FIFO Queue/1 -> #n/1
  Time-Based Function-Call Generator/1 -> Release Gate/1
  connections:
  FIFO Queue/RConn1 -- Release Gate/LConn1
  Release Gate/RConn1 -- Output/RConn1
  FIFO Queue/LConn1 -- Input/RConn1

== system Teste/Router2/Attribute Function ==
  MATLAB Function : MATLAB Function  TreatAsAtomicUnit=on
  __DMLF__EDE2FCE__ : EntityDepartureFunctionCallGenerator  TimingFunctionCallF1=Before entity departure  IsInsideAFB=on
  __DMLF__GA__ : GetAttribute  AttributeName=DST|ME  AttributeMissing=Error|Error  AttributeDefaultValue=1|1  AttributeTreatAsVector=1|1  AttributeSendTiming=Before entity departure|Before entity departure  EvaluatedDefaultAttributeValue={ [];[]}  IsInsideAFB=on
      settings: OutputPortMap=o1,o2
  __DMLF__SA__ : SetAttribute  AttributeName=RT  AttributeFrom=Signal port  EvaluatedAttributeValue={ []}  IsInsideAFB=on
  IN : PMIOPort  Side=Left
  OUT : PMIOPort  Port=2  Side=Right
  wires:
  MATLAB Function/1(out_RT) -> __DMLF__SA__/1
  __DMLF__GA__/2 -> MATLAB Function/2(ME)
  __DMLF__GA__/1 -> MATLAB Function/1(DST)
  __DMLF__EDE2FCE__/1 -> MATLAB Function/Trigger
  connections:
  __DMLF__SA__/RConn1 -- OUT/RConn1
  IN/RConn1 -- __DMLF__GA__/LConn1
  __DMLF__GA__/RConn1 -- __DMLF__EDE2FCE__/LConn1
  __DMLF__SA__/LConn1 -- __DMLF__EDE2FCE__/RConn1

== system Teste/Router2/Clocked FIFO1 ==
  Event-Based Random Number : EventBasedRandomNumber  Distribution=Gaussian (normal)  meanNorm=E  stdNorm=S
  FIFO Queue : FIFOQueue  Capacity=F  StatNumberInBlock=on
      settings: OutputPortMap=o1
  Release Gate : ReleaseGate  OpenGateUpon=Function call from port fcn
  Time-Based Function-Call Generator : TimeBasedFunctionCallGenerator  EventGenerationMode=Period from port  Period=T
  Input : PMIOPort  Side=Left
  Output : PMIOPort  Port=2  Side=Right
  #n : Outport
  wires:
  Event-Based Random Number/1 -> Time-Based Function-Call Generator/1
  FIFO Queue/1 -> #n/1
  Time-Based Function-Call Generator/1 -> Release Gate/1
  connections:
  FIFO Queue/RConn1 -- Release Gate/LConn1
  Release Gate/RConn1 -- Output/RConn1
  FIFO Queue/LConn1 -- Input/RConn1

== system Teste/Router2/Clocked FIFO2 ==
  Event-Based Random Number : EventBasedRandomNumber  Distribution=Gaussian (normal)  meanNorm=E  stdNorm=S
  FIFO Queue : FIFOQueue  Capacity=F  StatNumberInBlock=on
      settings: OutputPortMap=o1
  Release Gate : ReleaseGate  OpenGateUpon=Function call from port fcn
  Time-Based Function-Call Generator : TimeBasedFunctionCallGenerator  EventGenerationMode=Period from port  Period=T
  Input : PMIOPort  Side=Left
  Output : PMIOPort  Port=2  Side=Right
  #n : Outport
  wires:
  Event-Based Random Number/1 -> Time-Based Function-Call Generator/1
  FIFO Queue/1 -> #n/1
  Time-Based Function-Call Generator/1 -> Release Gate/1
  connections:
  FIFO Queue/RConn1 -- Release Gate/LConn1
  Release Gate/RConn1 -- Output/RConn1
  FIFO Queue/LConn1 -- Input/RConn1

== system Teste/Router2/Clocked FIFO3 ==
  Event-Based Random Number : EventBasedRandomNumber  Distribution=Gaussian (normal)  meanNorm=E  stdNorm=S
  FIFO Queue : FIFOQueue  Capacity=F  StatNumberInBlock=on
      settings: OutputPortMap=o1
  Release Gate : ReleaseGate  OpenGateUpon=Function call from port fcn
  Time-Based Function-Call Generator : TimeBasedFunctionCallGenerator  EventGenerationMode=Period from port  Period=T
  Input : PMIOPort  Side=Left
  Output : PMIOPort  Port=2  Side=Right
  #n : Outport
  wires:
  Event-Based Random Number/1 -> Time-Based Function-Call Generator/1
  FIFO Queue/1 -> #n/1
  Time-Based Function-Call Generator/1 -> Release Gate/1
  connections:
  FIFO Queue/RConn1 -- Release Gate/LConn1
  Release Gate/RConn1 -- Output/RConn1
  FIFO Queue/LConn1 -- Input/RConn1

== system Teste/Router2/Clocked FIFO4 ==
  Event-Based Random Number : EventBasedRandomNumber  Distribution=Gaussian (normal)  meanNorm=E  stdNorm=S
  FIFO Queue : FIFOQueue  Capacity=F  StatNumberInBlock=on
      settings: OutputPortMap=o1
  Release Gate : ReleaseGate  OpenGateUpon=Function call from port fcn
  Time-Based Function-Call Generator : TimeBasedFunctionCallGenerator  EventGenerationMode=Period from port  Period=T
  Input : PMIOPort  Side=Left
  Output : PMIOPort  Port=2  Side=Right
  #n : Outport
  wires:
  Event-Based Random Number/1 -> Time-Based Function-Call Generator/1
  FIFO Queue/1 -> #n/1
  Time-Based Function-Call Generator/1 -> Release Gate/1
  connections:
  FIFO Queue/RConn1 -- Release Gate/LConn1
  Release Gate/RConn1 -- Output/RConn1
  FIFO Queue/LConn1 -- Input/RConn1

== system Teste/Router2/Clocked FIFO5 ==
  Event-Based Random Number : EventBasedRandomNumber  Distribution=Gaussian (normal)  meanNorm=E  stdNorm=S
  FIFO Queue : FIFOQueue  Capacity=F  StatNumberInBlock=on
      settings: OutputPortMap=o1
  Release Gate : ReleaseGate  OpenGateUpon=Function call from port fcn
  Time-Based Function-Call Generator : TimeBasedFunctionCallGenerator  EventGenerationMode=Period from port  Period=T
  Input : PMIOPort  Side=Left
  Output : PMIOPort  Port=2  Side=Right
  #n : Outport
  wires:
  Event-Based Random Number/1 -> Time-Based Function-Call Generator/1
  FIFO Queue/1 -> #n/1
  Time-Based Function-Call Generator/1 -> Release Gate/1
  connections:
  FIFO Queue/RConn1 -- Release Gate/LConn1
  Release Gate/RConn1 -- Output/RConn1
  FIFO Queue/LConn1 -- Input/RConn1

== system Teste/Router3/Attribute Function ==
  MATLAB Function : MATLAB Function  TreatAsAtomicUnit=on
  __DMLF__EDE2FCE__ : EntityDepartureFunctionCallGenerator  TimingFunctionCallF1=Before entity departure  IsInsideAFB=on
  __DMLF__GA__ : GetAttribute  AttributeName=DST|ME  AttributeMissing=Error|Error  AttributeDefaultValue=1|1  AttributeTreatAsVector=1|1  AttributeSendTiming=Before entity departure|Before entity departure  EvaluatedDefaultAttributeValue={ [];[]}  IsInsideAFB=on
      settings: OutputPortMap=o1,o2
  __DMLF__SA__ : SetAttribute  AttributeName=RT  AttributeFrom=Signal port  EvaluatedAttributeValue={ []}  IsInsideAFB=on
  IN : PMIOPort  Side=Left
  OUT : PMIOPort  Port=2  Side=Right
  wires:
  MATLAB Function/1(out_RT) -> __DMLF__SA__/1
  __DMLF__GA__/2 -> MATLAB Function/2(ME)
  __DMLF__GA__/1 -> MATLAB Function/1(DST)
  __DMLF__EDE2FCE__/1 -> MATLAB Function/Trigger
  connections:
  __DMLF__SA__/RConn1 -- OUT/RConn1
  IN/RConn1 -- __DMLF__GA__/LConn1
  __DMLF__GA__/RConn1 -- __DMLF__EDE2FCE__/LConn1
  __DMLF__SA__/LConn1 -- __DMLF__EDE2FCE__/RConn1

== system Teste/Router3/Clocked FIFO1 ==
  Event-Based Random Number : EventBasedRandomNumber  Distribution=Gaussian (normal)  meanNorm=E  stdNorm=S
  FIFO Queue : FIFOQueue  Capacity=F  StatNumberInBlock=on
      settings: OutputPortMap=o1
  Release Gate : ReleaseGate  OpenGateUpon=Function call from port fcn
  Time-Based Function-Call Generator : TimeBasedFunctionCallGenerator  EventGenerationMode=Period from port  Period=T
  Input : PMIOPort  Side=Left
  Output : PMIOPort  Port=2  Side=Right
  #n : Outport
  wires:
  Event-Based Random Number/1 -> Time-Based Function-Call Generator/1
  FIFO Queue/1 -> #n/1
  Time-Based Function-Call Generator/1 -> Release Gate/1
  connections:
  FIFO Queue/RConn1 -- Release Gate/LConn1
  Release Gate/RConn1 -- Output/RConn1
  FIFO Queue/LConn1 -- Input/RConn1

== system Teste/Router3/Clocked FIFO2 ==
  Event-Based Random Number : EventBasedRandomNumber  Distribution=Gaussian (normal)  meanNorm=E  stdNorm=S
  FIFO Queue : FIFOQueue  Capacity=F  StatNumberInBlock=on
      settings: OutputPortMap=o1
  Release Gate : ReleaseGate  OpenGateUpon=Function call from port fcn
  Time-Based Function-Call Generator : TimeBasedFunctionCallGenerator  EventGenerationMode=Period from port  Period=T
  Input : PMIOPort  Side=Left
  Output : PMIOPort  Port=2  Side=Right
  #n : Outport
  wires:
  Event-Based Random Number/1 -> Time-Based Function-Call Generator/1
  FIFO Queue/1 -> #n/1
  Time-Based Function-Call Generator/1 -> Release Gate/1
  connections:
  FIFO Queue/RConn1 -- Release Gate/LConn1
  Release Gate/RConn1 -- Output/RConn1
  FIFO Queue/LConn1 -- Input/RConn1

== system Teste/Router3/Clocked FIFO3 ==
  Event-Based Random Number : EventBasedRandomNumber  Distribution=Gaussian (normal)  meanNorm=E  stdNorm=S
  FIFO Queue : FIFOQueue  Capacity=F  StatNumberInBlock=on
      settings: OutputPortMap=o1
  Release Gate : ReleaseGate  OpenGateUpon=Function call from port fcn
  Time-Based Function-Call Generator : TimeBasedFunctionCallGenerator  EventGenerationMode=Period from port  Period=T
  Input : PMIOPort  Side=Left
  Output : PMIOPort  Port=2  Side=Right
  #n : Outport
  wires:
  Event-Based Random Number/1 -> Time-Based Function-Call Generator/1
  FIFO Queue/1 -> #n/1
  Time-Based Function-Call Generator/1 -> Release Gate/1
  connections:
  FIFO Queue/RConn1 -- Release Gate/LConn1
  Release Gate/RConn1 -- Output/RConn1
  FIFO Queue/LConn1 -- Input/RConn1

== system Teste/Router3/Clocked FIFO4 ==
  Event-Based Random Number : EventBasedRandomNumber  Distribution=Gaussian (normal)  meanNorm=E  stdNorm=S
  FIFO Queue : FIFOQueue  Capacity=F  StatNumberInBlock=on
      settings: OutputPortMap=o1
  Release Gate : ReleaseGate  OpenGateUpon=Function call from port fcn
  Time-Based Function-Call Generator : TimeBasedFunctionCallGenerator  EventGenerationMode=Period from port  Period=T
  Input : PMIOPort  Side=Left
  Output : PMIOPort  Port=2  Side=Right
  #n : Outport
  wires:
  Event-Based Random Number/1 -> Time-Based Function-Call Generator/1
  FIFO Queue/1 -> #n/1
  Time-Based Function-Call Generator/1 -> Release Gate/1
  connections:
  FIFO Queue/RConn1 -- Release Gate/LConn1
  Release Gate/RConn1 -- Output/RConn1
  FIFO Queue/LConn1 -- Input/RConn1

== system Teste/Router3/Clocked FIFO5 ==
  Event-Based Random Number : EventBasedRandomNumber  Distribution=Gaussian (normal)  meanNorm=E  stdNorm=S
  FIFO Queue : FIFOQueue  Capacity=F  StatNumberInBlock=on
      settings: OutputPortMap=o1
  Release Gate : ReleaseGate  OpenGateUpon=Function call from port fcn
  Time-Based Function-Call Generator : TimeBasedFunctionCallGenerator  EventGenerationMode=Period from port  Period=T
  Input : PMIOPort  Side=Left
  Output : PMIOPort  Port=2  Side=Right
  #n : Outport
  wires:
  Event-Based Random Number/1 -> Time-Based Function-Call Generator/1
  FIFO Queue/1 -> #n/1
  Time-Based Function-Call Generator/1 -> Release Gate/1
  connections:
  FIFO Queue/RConn1 -- Release Gate/LConn1
  Release Gate/RConn1 -- Output/RConn1
  FIFO Queue/LConn1 -- Input/RConn1

== system Teste/Router4/Attribute Function ==
  MATLAB Function : MATLAB Function  TreatAsAtomicUnit=on
  __DMLF__EDE2FCE__ : EntityDepartureFunctionCallGenerator  TimingFunctionCallF1=Before entity departure  IsInsideAFB=on
  __DMLF__GA__ : GetAttribute  AttributeName=DST|ME  AttributeMissing=Error|Error  AttributeDefaultValue=1|1  AttributeTreatAsVector=1|1  AttributeSendTiming=Before entity departure|Before entity departure  EvaluatedDefaultAttributeValue={ [];[]}  IsInsideAFB=on
      settings: OutputPortMap=o1,o2
  __DMLF__SA__ : SetAttribute  AttributeName=RT  AttributeFrom=Signal port  EvaluatedAttributeValue={ []}  IsInsideAFB=on
  IN : PMIOPort  Side=Left
  OUT : PMIOPort  Port=2  Side=Right
  wires:
  MATLAB Function/1(out_RT) -> __DMLF__SA__/1
  __DMLF__GA__/2 -> MATLAB Function/2(ME)
  __DMLF__GA__/1 -> MATLAB Function/1(DST)
  __DMLF__EDE2FCE__/1 -> MATLAB Function/Trigger
  connections:
  __DMLF__SA__/RConn1 -- OUT/RConn1
  IN/RConn1 -- __DMLF__GA__/LConn1
  __DMLF__GA__/RConn1 -- __DMLF__EDE2FCE__/LConn1
  __DMLF__SA__/LConn1 -- __DMLF__EDE2FCE__/RConn1

== system Teste/Router4/Clocked FIFO1 ==
  Event-Based Random Number : EventBasedRandomNumber  Distribution=Gaussian (normal)  meanNorm=E  stdNorm=S
  FIFO Queue : FIFOQueue  Capacity=F  StatNumberInBlock=on
      settings: OutputPortMap=o1
  Release Gate : ReleaseGate  OpenGateUpon=Function call from port fcn
  Time-Based Function-Call Generator : TimeBasedFunctionCallGenerator  EventGenerationMode=Period from port  Period=T
  Input : PMIOPort  Side=Left
  Output : PMIOPort  Port=2  Side=Right
  #n : Outport
  wires:
  Event-Based Random Number/1 -> Time-Based Function-Call Generator/1
  FIFO Queue/1 -> #n/1
  Time-Based Function-Call Generator/1 -> Release Gate/1
  connections:
  FIFO Queue/RConn1 -- Release Gate/LConn1
  Release Gate/RConn1 -- Output/RConn1
  FIFO Queue/LConn1 -- Input/RConn1

== system Teste/Router4/Clocked FIFO2 ==
  Event-Based Random Number : EventBasedRandomNumber  Distribution=Gaussian (normal)  meanNorm=E  stdNorm=S
  FIFO Queue : FIFOQueue  Capacity=F  StatNumberInBlock=on
      settings: OutputPortMap=o1
  Release Gate : ReleaseGate  OpenGateUpon=Function call from port fcn
  Time-Based Function-Call Generator : TimeBasedFunctionCallGenerator  EventGenerationMode=Period from port  Period=T
  Input : PMIOPort  Side=Left
  Output : PMIOPort  Port=2  Side=Right
  #n : Outport
  wires:
  Event-Based Random Number/1 -> Time-Based Function-Call Generator/1
  FIFO Queue/1 -> #n/1
  Time-Based Function-Call Generator/1 -> Release Gate/1
  connections:
  FIFO Queue/RConn1 -- Release Gate/LConn1
  Release Gate/RConn1 -- Output/RConn1
  FIFO Queue/LConn1 -- Input/RConn1

== system Teste/Router4/Clocked FIFO3 ==
  Event-Based Random Number : EventBasedRandomNumber  Distribution=Gaussian (normal)  meanNorm=E  stdNorm=S
  FIFO Queue : FIFOQueue  Capacity=F  StatNumberInBlock=on
      settings: OutputPortMap=o1
  Release Gate : ReleaseGate  OpenGateUpon=Function call from port fcn
  Time-Based Function-Call Generator : TimeBasedFunctionCallGenerator  EventGenerationMode=Period from port  Period=T
  Input : PMIOPort  Side=Left
  Output : PMIOPort  Port=2  Side=Right
  #n : Outport
  wires:
  Event-Based Random Number/1 -> Time-Based Function-Call Generator/1
  FIFO Queue/1 -> #n/1
  Time-Based Function-Call Generator/1 -> Release Gate/1
  connections:
  FIFO Queue/RConn1 -- Release Gate/LConn1
  Release Gate/RConn1 -- Output/RConn1
  FIFO Queue/LConn1 -- Input/RConn1

== system Teste/Router4/Clocked FIFO4 ==
  Event-Based Random Number : EventBasedRandomNumber  Distribution=Gaussian (normal)  meanNorm=E  stdNorm=S
  FIFO Queue : FIFOQueue  Capacity=F  StatNumberInBlock=on
      settings: OutputPortMap=o1
  Release Gate : ReleaseGate  OpenGateUpon=Function call from port fcn
  Time-Based Function-Call Generator : TimeBasedFunctionCallGenerator  EventGenerationMode=Period from port  Period=T
  Input : PMIOPort  Side=Left
  Output : PMIOPort  Port=2  Side=Right
  #n : Outport
  wires:
  Event-Based Random Number/1 -> Time-Based Function-Call Generator/1
  FIFO Queue/1 -> #n/1
  Time-Based Function-Call Generator/1 -> Release Gate/1
  connections:
  FIFO Queue/RConn1 -- Release Gate/LConn1
  Release Gate/RConn1 -- Output/RConn1
  FIFO Queue/LConn1 -- Input/RConn1

== system Teste/Router4/Clocked FIFO5 ==
  Event-Based Random Number : EventBasedRandomNumber  Distribution=Gaussian (normal)  meanNorm=E  stdNorm=S
  FIFO Queue : FIFOQueue  Capacity=F  StatNumberInBlock=on
      settings: OutputPortMap=o1
  Release Gate : ReleaseGate  OpenGateUpon=Function call from port fcn
  Time-Based Function-Call Generator : TimeBasedFunctionCallGenerator  EventGenerationMode=Period from port  Period=T
  Input : PMIOPort  Side=Left
  Output : PMIOPort  Port=2  Side=Right
  #n : Outport
  wires:
  Event-Based Random Number/1 -> Time-Based Function-Call Generator/1
  FIFO Queue/1 -> #n/1
  Time-Based Function-Call Generator/1 -> Release Gate/1
  connections:
  FIFO Queue/RConn1 -- Release Gate/LConn1
  Release Gate/RConn1 -- Output/RConn1
  FIFO Queue/LConn1 -- Input/RConn1

== system Teste/Router5/Attribute Function ==
  MATLAB Function : MATLAB Function  TreatAsAtomicUnit=on
  __DMLF__EDE2FCE__ : EntityDepartureFunctionCallGenerator  TimingFunctionCallF1=Before entity departure  IsInsideAFB=on
  __DMLF__GA__ : GetAttribute  AttributeName=DST|ME  AttributeMissing=Error|Error  AttributeDefaultValue=1|1  AttributeTreatAsVector=1|1  AttributeSendTiming=Before entity departure|Before entity departure  EvaluatedDefaultAttributeValue={ [];[]}  IsInsideAFB=on
      settings: OutputPortMap=o1,o2
  __DMLF__SA__ : SetAttribute  AttributeName=RT  AttributeFrom=Signal port  EvaluatedAttributeValue={ []}  IsInsideAFB=on
  IN : PMIOPort  Side=Left
  OUT : PMIOPort  Port=2  Side=Right
  wires:
  MATLAB Function/1(out_RT) -> __DMLF__SA__/1
  __DMLF__GA__/2 -> MATLAB Function/2(ME)
  __DMLF__GA__/1 -> MATLAB Function/1(DST)
  __DMLF__EDE2FCE__/1 -> MATLAB Function/Trigger
  connections:
  __DMLF__SA__/RConn1 -- OUT/RConn1
  IN/RConn1 -- __DMLF__GA__/LConn1
  __DMLF__GA__/RConn1 -- __DMLF__EDE2FCE__/LConn1
  __DMLF__SA__/LConn1 -- __DMLF__EDE2FCE__/RConn1
